simulink model "auv_sonar_waveform_pipeline"  (R2026a)
settings: Solver=FixedStepDiscrete  StopTime=Tp  FixedStep=Ts_dac
PreLoadFcn:
  | % Self-healing path configuration for AUV Sonar Simulink Suite
  | m_file = get_param(bdroot, 'FileName');
  | if ~isempty(m_file)
  |     m_dir = fileparts(m_file);
  |     addpath(m_dir);
  |     addpath(fullfile(m_dir, '..'));
  | else
  |     if exist(fullfile(pwd, 'matlab', 'simulink'), 'dir')
  |         addpath(fullfile(pwd, 'matlab', 'simulink'));
  |         addpath(fullfile(pwd, 'matlab'));
  |     end
  | end
  | if exist('init_sonar_simulink', 'file') == 2
  |     init_sonar_simulink;
  | end
InitFcn:
  | % Self-healing path configuration for AUV Sonar Simulink Suite
  | m_file = get_param(bdroot, 'FileName');
  | if ~isempty(m_file)
  |     m_dir = fileparts(m_file);
  |     addpath(m_dir);
  |     addpath(fullfile(m_dir, '..'));
  | else
  |     if exist(fullfile(pwd, 'matlab', 'simulink'), 'dir')
  |         addpath(fullfile(pwd, 'matlab', 'simulink'));
  |         addpath(fullfile(pwd, 'matlab'));
  |     end
  | end
  | if exist('init_sonar_simulink', 'file') == 2
  |     init_sonar_simulink;
  | end
undefined symbols (not defined in the file or in its folder): Ts_dac
settings Model: Creator=harsh  LastModifiedBy=harsh

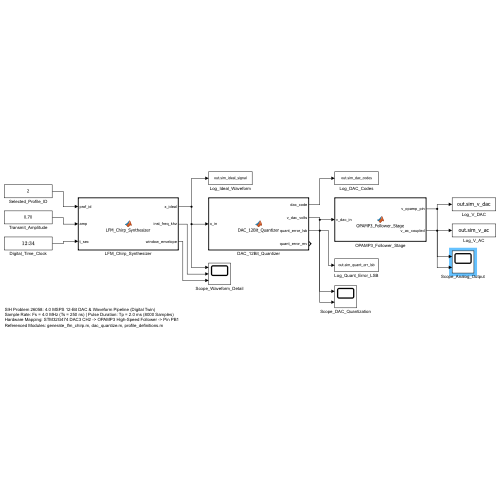
[thumbnail: Simulink's stored preview of the top-level diagram]
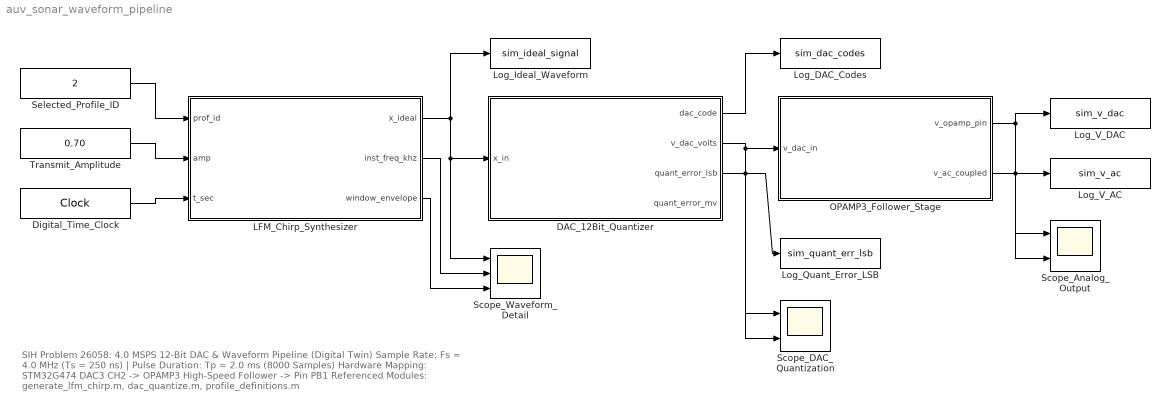
== system auv_sonar_waveform_pipeline ==
  note: SIH Problem 26058: 4.0 MSPS 12-Bit DAC & Waveform Pipeline (Digital Twin)
      | Sample Rate: Fs = 4.0 MHz (Ts = 250 ns) | Pulse Duration: Tp = 2.0 ms (8000 Samples)
      | Hardware Mapping: STM32G474 DAC3 CH2 -> OPAMP3 High-Speed Follower -> Pin PB1
      | Referenced Modules: generate_lfm_chirp.m, dac_quantize.m, profile_definitions.m
  DAC_12Bit_Quantizer : MATLAB Function  TreatAsAtomicUnit=on
  Digital_Time_Clock : DigitalClock  SampleTime=Ts_dac
  LFM_Chirp_Synthesizer : MATLAB Function  TreatAsAtomicUnit=on
  Log_DAC_Codes : ToWorkspace  VariableName=sim_dac_codes  SampleTime=-1
  Log_Ideal_Waveform : ToWorkspace  VariableName=sim_ideal_signal  SampleTime=-1
  Log_Quant_Error_LSB : ToWorkspace  VariableName=sim_quant_err_lsb  SampleTime=-1
  Log_V_AC : ToWorkspace  VariableName=sim_v_ac  SampleTime=-1
  Log_V_DAC : ToWorkspace  VariableName=sim_v_dac  SampleTime=-1
  OPAMP3_Follower_Stage : MATLAB Function  TreatAsAtomicUnit=on
  Scope_Analog_Output : Scope  NumInputPorts=2
      settings: ActiveDisplayYMinimum=-5.0828975603709843  ActiveDisplayYMaximum=4.91886334058492
  Scope_DAC_Quantization : Scope  NumInputPorts=2
      settings: ActiveDisplayYMinimum=-3.7427231208663283  ActiveDisplayYMaximum=4.8463717049765247
  Scope_Waveform_Detail : Scope  NumInputPorts=3
      settings: ActiveDisplayYMinimum=-556.3938259300337  ActiveDisplayYMaximum=772.5764473266845
  Selected_Profile_ID : Constant  Value=2  SampleTime=Ts_dac
  Transmit_Amplitude : Constant  Value=0.70  SampleTime=Ts_dac
  wires:
  Selected_Profile_ID/1 -> LFM_Chirp_Synthesizer/1(prof_id)
  Transmit_Amplitude/1 -> LFM_Chirp_Synthesizer/2(amp)
  Digital_Time_Clock/1 -> LFM_Chirp_Synthesizer/3(t_sec)
  LFM_Chirp_Synthesizer/1(x_ideal) -> DAC_12Bit_Quantizer/1(x_in), Scope_Waveform_Detail/1, Log_Ideal_Waveform/1
  LFM_Chirp_Synthesizer/2(inst_freq_khz) -> Scope_Waveform_Detail/2
  LFM_Chirp_Synthesizer/3(window_envelope) -> Scope_Waveform_Detail/3
  DAC_12Bit_Quantizer/1(dac_code) -> Log_DAC_Codes/1
  DAC_12Bit_Quantizer/2(v_dac_volts) -> OPAMP3_Follower_Stage/1(v_dac_in), Scope_DAC_Quantization/1
  DAC_12Bit_Quantizer/3(quant_error_lsb) -> Log_Quant_Error_LSB/1, Scope_DAC_Quantization/2
  OPAMP3_Follower_Stage/1(v_opamp_pin) -> Log_V_DAC/1, Scope_Analog_Output/1
  OPAMP3_Follower_Stage/2(v_ac_coupled) -> Log_V_AC/1, Scope_Analog_Output/2

== matlab function auv_sonar_waveform_pipeline/DAC_12Bit_Quantizer ==
  data: x_in input; dac_code output; v_dac_volts output; quant_error_lsb output; quant_error_mv output
function [dac_code, v_dac_volts, quant_error_lsb, quant_error_mv] = DAC_12Bit_Quantizer(x_in)
coder.extrinsic('sim_bridge_dac');
dac_code = 2048.0;
v_dac_volts = 1.65;
quant_error_lsb = 0.0;
quant_error_mv = 0.0;
[dac_code, v_dac_volts, quant_error_lsb, quant_error_mv] = sim_bridge_dac(x_in);
end

== matlab function auv_sonar_waveform_pipeline/LFM_Chirp_Synthesizer ==
  data: prof_id input; x_ideal output; amp input; t_sec input; inst_freq_khz output; window_envelope output
function [x_ideal, inst_freq_khz, window_envelope] = LFM_Chirp_Synthesizer(prof_id, amp, t_sec)
coder.extrinsic('sim_bridge_waveform');
x_ideal = 0.0;
inst_freq_khz = 200.0;
window_envelope = 0.0;
[x_ideal, inst_freq_khz, window_envelope] = sim_bridge_waveform(prof_id, amp, t_sec);
end

== matlab function auv_sonar_waveform_pipeline/OPAMP3_Follower_Stage ==
  data: v_dac_in input; v_opamp_pin output; v_ac_coupled output
function [v_opamp_pin, v_ac_coupled] = OPAMP3_Follower_Stage(v_dac_in)
v_opamp_pin = max(0.0, min(3.3, v_dac_in));
v_ac_coupled = v_opamp_pin - 1.65;
end
